simulink model "discrete_unscented_kalman"  (R2015b)
settings: Solver=VariableStepAuto  StartTime=0.0  StopTime=10.0  RelTol=1e-3
settings Model: Creator=mgreiff  LastModifiedBy=mgreiff

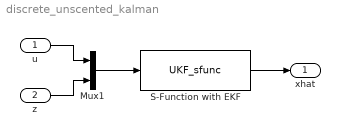
== system discrete_unscented_kalman ==
  u : Inport  PortDimensions=4
  z : Inport  Port=2  PortDimensions=9
  Mux1 : Mux  Inputs=2
  S-Function with EKF : S-Function  FunctionName=UKF_sfunc  Parameters=KFparam  SFunctionDeploymentMode=off  EnableBusSupport=off
  xhat : Outport
  wires:
  u/1 -> Mux1/1
  z/1 -> Mux1/2
  S-Function with EKF/1 -> xhat/1
  Mux1/1 -> S-Function with EKF/1
